simulink model "CRIT4INDIstab"  (R2019b)
settings: Solver=VariableStepAuto  StartTime=0.0  StopTime=10.0  RelTol=1e-3
values from neighbouring files (symbols this model uses):
  Ah3 = blkdiag(Ah3, Ahc)    [HinFSynINDIstab.m]
  Ah7 = blkdiag(Ah7, Ahc)    [HinFSynINDIstab.m]
  Amc = d2c(Amd,'tustin')    [HinFSynINDIstab.m]
  Asc = d2c(Asd,'tustin')    [HinFSynINDIstab.m]
  Bh3 = blkdiag(Bh3, Bhc)    [HinFSynINDIstab.m]
  Bh7 = blkdiag(Bh7, Bhc)    [HinFSynINDIstab.m]
  Ch3 = blkdiag(Ch3, Chc)    [HinFSynINDIstab.m]
  Ch7 = blkdiag(Ch7, Chc)    [HinFSynINDIstab.m]
  Dh3 = blkdiag(Dh3, Dhc)    [HinFSynINDIstab.m]
  Dh7 = blkdiag(Dh7, Dhc)    [HinFSynINDIstab.m]
  G = [-10.67  10.67  0     0     0     0 0 ... (first row only)    [HinFSynINDIstab.m]
  G_inv = pinv(G)    [HinFSynINDIstab.m]
  G_thrust = [0 0 0 0 0 0 0 ... (first row only)    [HinFSynINDIstab.m]
  Kd = [10; 18; 18]    [HinFSynINDIstab.m]
  Kp = blkdiag(Kroll.D,Kpitch.D,Kyaw.D)    [HinFSynINDIstab.m]
settings Model: Creator=demouran  LastModifiedBy=demouran

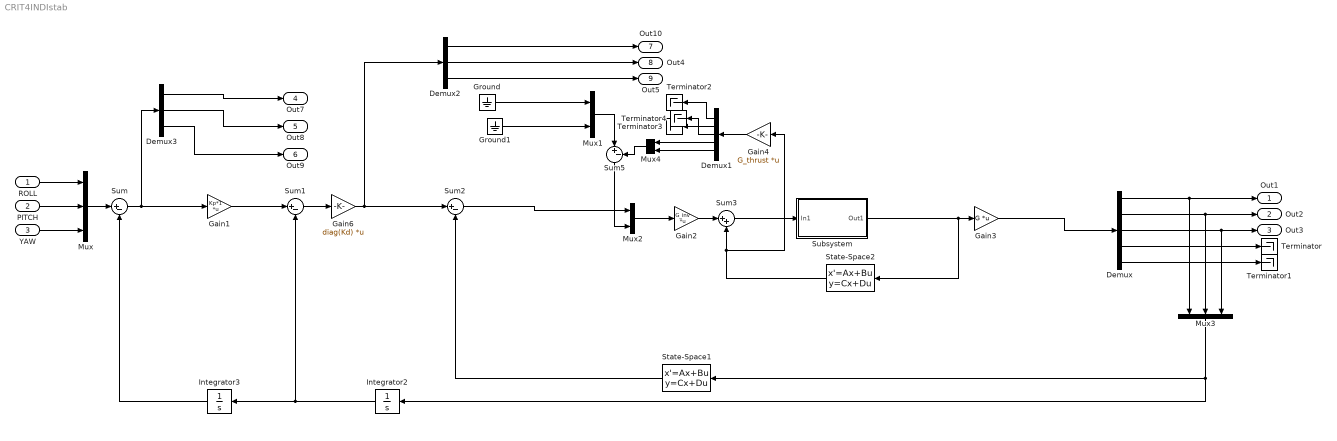
== system CRIT4INDIstab ==
  ROLL : Inport
  PITCH : Inport  Port=2
  YAW : Inport  Port=3
  Demux : Demux  Outputs=5
  Demux1 : Demux  Outputs=5
  Demux2 : Demux  Outputs=3
  Demux3 : Demux  Outputs=3
  Gain1 : Gain  Gain=Kp*1  Multiplication=Matrix(K*u)
  Gain2 : Gain  Gain=G_inv  Multiplication=Matrix(K*u)
  Gain3 : Gain  Gain=G  Multiplication=Matrix(K*u)
  Gain4 : Gain  Gain=G_thrust  Multiplication=Matrix(K*u)
  Gain6 : Gain  Gain=diag(Kd)  Multiplication=Matrix(K*u)
  Ground : Ground
  Ground1 : Ground
  Integrator2 : Integrator
  Integrator3 : Integrator
  Mux : Mux  Inputs=3
  Mux1 : Mux  Inputs=2
  Mux2 : Mux  Inputs=[3 2]
  Mux3 : Mux  Inputs=3
  Mux4 : Mux  Inputs=2
  State-Space1 : StateSpace  A=Ah3  B=Bh3  C=Ch3  D=Dh3  InitialCondition=0
  State-Space2 : StateSpace  A=Ah7  B=Bh7  C=Ch7  D=Dh7  InitialCondition=0
  Subsystem : Subsystem
  Sum{,1..2,5} (4 alike) : Sum  Inputs=|+-
  Sum3 : Sum  Inputs=|++
  Terminator{,1..4} (5 alike) : Terminator
  Out1 : Outport
  Out2 : Outport  Port=2
  Out3 : Outport  Port=3
  Out7 : Outport  Port=4
  Out8 : Outport  Port=5
  Out9 : Outport  Port=6
  Out10 : Outport  Port=7
  Out4 : Outport  Port=8
  Out5 : Outport  Port=9
  wires:
  Demux/5 -> Terminator1/1
  Demux/4 -> Terminator/1
  Demux/3 -> Out3/1, Mux3/3
  Demux/2 -> Out2/1, Mux3/2
  Demux/1 -> Out1/1, Mux3/1
  Integrator2/1 -> Sum1/2, Integrator3/1
  Sum1/1 -> Gain6/1
  Gain1/1 -> Sum1/1
  Integrator3/1 -> Sum/2
  Demux3/2 -> Out8/1
  Demux3/3 -> Out9/1
  Demux2/1 -> Out10/1
  Demux2/2 -> Out4/1
  Demux2/3 -> Out5/1
  ROLL/1 -> Mux/1
  PITCH/1 -> Mux/2
  YAW/1 -> Mux/3
  Mux/1 -> Sum/1
  Sum/1 -> Gain1/1, Demux3/1
  Gain3/1 -> Demux/1
  Sum3/1 -> Subsystem/1(In1)
  Gain2/1 -> Sum3/1
  Gain6/1 -> Sum2/1, Demux2/1
  State-Space1/1 -> Sum2/2
  Mux3/1 -> State-Space1/1, Integrator2/1
  Mux2/1 -> Gain2/1
  Sum2/1 -> Mux2/1
  Subsystem/1(Out1) -> State-Space2/1, Gain3/1
  Demux1/3 -> Terminator4/1
  Mux1/1 -> Sum5/1
  Demux1/4 -> Mux4/1
  Demux1/2 -> Terminator3/1
  State-Space2/1 -> Gain4/1, Sum3/2
  Mux4/1 -> Sum5/2
  Demux1/1 -> Terminator2/1
  Demux1/5 -> Mux4/2
  Sum5/1 -> Mux2/2
  Gain4/1 -> Demux1/1
  Ground/1 -> Mux1/1
  Ground1/1 -> Mux1/2
  Demux3/1 -> Out7/1

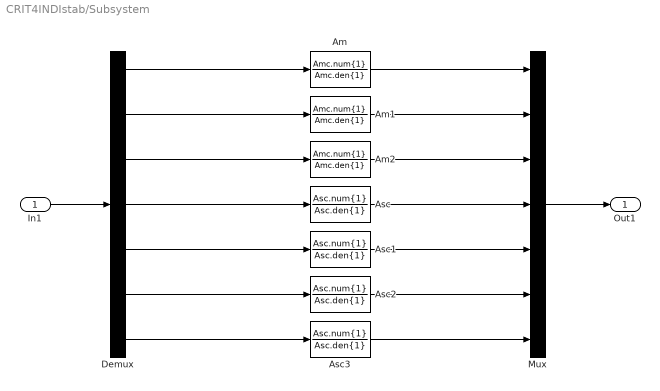
== system CRIT4INDIstab/Subsystem ==
  In1 : Inport
  Am : TransferFcn  Numerator=Amc.num{1}  Denominator=Amc.den{1}
  Am1 : TransferFcn  Numerator=Amc.num{1}  Denominator=Amc.den{1}
  Am2 : TransferFcn  Numerator=Amc.num{1}  Denominator=Amc.den{1}
  Asc{,1..3} (4 alike) : TransferFcn  Numerator=Asc.num{1}  Denominator=Asc.den{1}
  Demux : Demux  Outputs=7
  Mux : Mux  Inputs=7
  Out1 : Outport
  wires:
  Demux/5 -> Asc1/1
  Asc/1 -> Mux/4
  Demux/4 -> Asc/1
  Asc1/1 -> Mux/5
  Asc2/1 -> Mux/6
  Demux/6 -> Asc2/1
  Asc3/1 -> Mux/7
  Demux/7 -> Asc3/1
  In1/1 -> Demux/1
  Mux/1 -> Out1/1
  Demux/1 -> Am/1
  Am/1 -> Mux/1
  Am1/1 -> Mux/2
  Demux/2 -> Am1/1
  Am2/1 -> Mux/3
  Demux/3 -> Am2/1
